simulink model "cxfpid_part2_ant"  (Simulink 7.6)
settings: Solver=ode15s  StartTime=0.0  StopTime=100  RelTol=1e-3
PreLoadFcn:
  | L=1; M=1;
undefined symbols (not defined in the file or in its folder): Kd2, Ki2, Kp2, L2, M2
settings Model: Creator=Professor Dingyu Xue  LastModifiedBy=Pragya
settings OptimizationCC: InitFltsAndDblsToZero=on
settings DebuggingCC: SolverPrmCheckMsg=none  StrictBusMsg=Warning

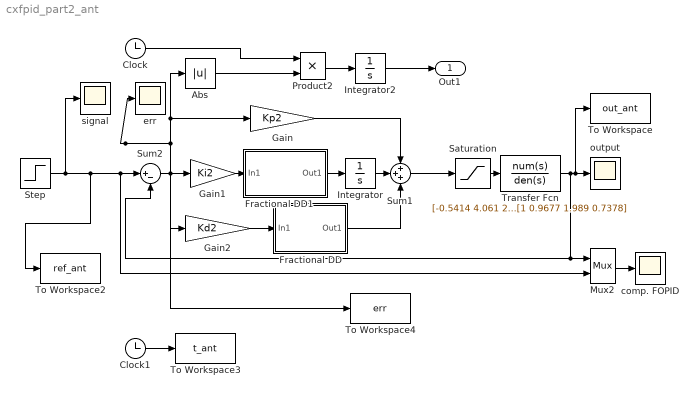
== system cxfpid_part2_ant ==
  Abs : Abs
  Clock : Clock
      settings: Decimation=10
  Clock1 : Clock
      settings: Decimation=10
  Fractional DD : Subsystem  mask{gam=M2, ww=[1e-3 1e3], n=2, key=Oustaloup's filter}
      mask prompts: gam "Derivative order gamma"; ww "Frequency range [wb,wh]"; n "Apprixmation order"; key "Selected filter"
      mask help: Fractional-order differentiator with Oustaloup's or modified Oustaloup's filter. The fitting frequency range and order should also be specified.
      mask init:
      | wb=ww(1); wh=ww(2); 
      | if key==1, G=ousta_fod(gam,n,wb,wh);
      | else, G=tf(new_fod(gam,n,wb,wh)); end
      | num=G.num{1}; den=G.den{1}; T=1/wh; str='Fractional\n';
      | if isnumeric(gam)
      | 	if gam>0, str=[str, 'Der  s^' num2str(0.01*round(100*gam)) ];
      | 	else, str=[str, 'Int  s^{' num2str(0.01*round(100*gam)) '}']; end
      | else, str=[str, 'Der  s^gam']; end
      mask StyleString: edit,edit,edit,popup(Oustaloup's filter|Modified Oustaloup's filter )
      mask Display: disp(str)
  Fractional DD1 : Subsystem  mask{gam=L2, ww=[1e-3 1e3], n=2, key=Oustaloup's filter}
      mask prompts: gam "Derivative order gamma"; ww "Frequency range [wb,wh]"; n "Apprixmation order"; key "Selected filter"
      mask help: Fractional-order differentiator with Oustaloup's or modified Oustaloup's filter. The fitting frequency range and order should also be specified.
      mask init: same as cxfpid_part2_ant/Fractional DD
      mask StyleString: edit,edit,edit,popup(Oustaloup's filter|Modified Oustaloup's filter )
      mask Display: disp(str)
  Gain : Gain  Gain=Kp2
  Gain1 : Gain  Gain=Ki2
  Gain2 : Gain  Gain=Kd2
  Integrator : Integrator
  Integrator2 : Integrator
  Mux2 : Mux  Inputs=2
  Product2 : Product  RndMeth=Zero
  Saturation : Saturate  UpperLimit=2  LowerLimit=-2
  Step : Step  Time=0  SampleTime=0
  Sum1 : Sum  Inputs=+++
  Sum2 : Sum  Inputs=|+-
  To Workspace : ToWorkspace  VariableName=out_ant  SampleTime=-1  SaveFormat=Array
  To Workspace2 : ToWorkspace  VariableName=ref_ant  SampleTime=-1  SaveFormat=Array
  To Workspace3 : ToWorkspace  VariableName=t_ant  SampleTime=-1  SaveFormat=Array
  To Workspace4 : ToWorkspace  VariableName=err  SampleTime=-1  SaveFormat=Array
  Transfer Fcn : TransferFcn  Numerator=[-0.5414 4.061 2.945]  Denominator=[1 0.9677 1.989 0.7378]
  comp. FOPID : Scope
      settings: TickLabels=on  TimeRange=10  YMin=0  YMax=2.1  SaveName=dc_pid1  DataFormat=Array
  err : Scope
      settings: TimeRange=15  YMin=1.23519  YMax=1.36521  SaveName=yy1  DataFormat=Array
  output : Scope
      settings: TickLabels=on  TimeRange=10  YMin=0.25  YMax=1.75  SaveName=fopid  DataFormat=Array
  signal : Scope
      settings: TickLabels=on  TimeRange=100  YMin=1.23519  YMax=1.36521  SaveName=sig  DataFormat=Array
  Out1 : Outport
  wires:
  Gain/1 -> Sum1/1
  Fractional DD/1(Out1) -> Sum1/3
  Gain1/1 -> Fractional DD1/1(In1)
  Gain2/1 -> Fractional DD/1(In1)
  Sum2/1 -> Gain/1, Abs/1, err/1, To Workspace4/1, Gain1/1, Gain2/1
  Transfer Fcn/1 -> Sum2/2, Mux2/1, output/1, To Workspace/1
  Mux2/1 -> comp. FOPID/1
  Integrator/1 -> Sum1/2
  Fractional DD1/1(Out1) -> Integrator/1
  Integrator2/1 -> Out1/1
  Abs/1 -> Product2/2
  Clock/1 -> Product2/1
  Product2/1 -> Integrator2/1
  Step/1 -> signal/1, Sum2/1, Mux2/2, To Workspace2/1
  Sum1/1 -> Saturation/1
  Saturation/1 -> Transfer Fcn/1
  Clock1/1 -> To Workspace3/1

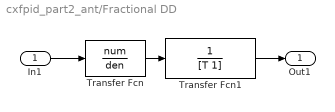
== system cxfpid_part2_ant/Fractional DD ==
  In1 : Inport
  Transfer Fcn : TransferFcn  Numerator=num  Denominator=den
  Transfer Fcn1 : TransferFcn  Numerator=1  Denominator=[T 1]
  Out1 : Outport
  wires:
  In1/1 -> Transfer Fcn/1
  Transfer Fcn/1 -> Transfer Fcn1/1
  Transfer Fcn1/1 -> Out1/1

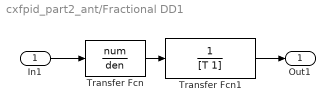
== system cxfpid_part2_ant/Fractional DD1 ==
  In1 : Inport
  Transfer Fcn : TransferFcn  Numerator=num  Denominator=den
  Transfer Fcn1 : TransferFcn  Numerator=1  Denominator=[T 1]
  Out1 : Outport
  wires:
  Transfer Fcn1/1 -> Out1/1
  Transfer Fcn/1 -> Transfer Fcn1/1
  In1/1 -> Transfer Fcn/1
